simulink model "simulink10_3"  (R2025b)
settings: Solver=ode45  StartTime=0.0  StopTime=150.0  MaxStep=0.05  RelTol=1e-3
values from neighbouring files (symbols this model uses):
  C = Rs*Ps^-1    [lab10.m]
undefined symbols (not defined in the file or in its folder): A, B, D
settings Model: Creator=mizula  LastModifiedBy=mizula

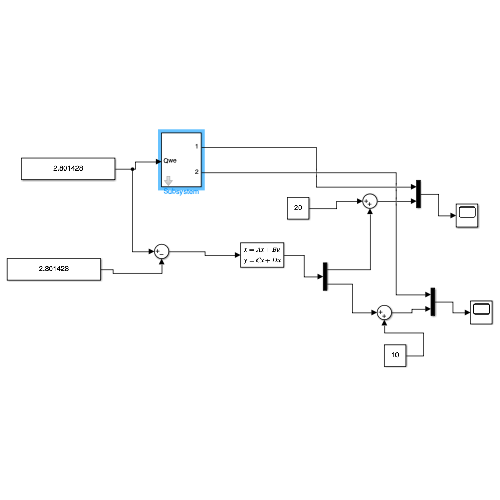
[thumbnail: Simulink's stored preview of the top-level diagram]
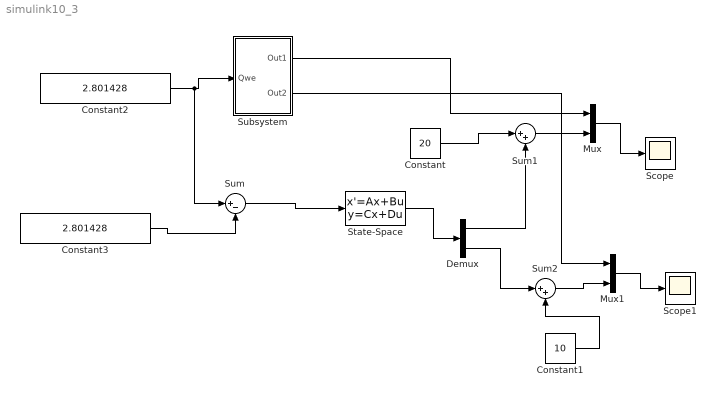
== system simulink10_3 ==
  Constant : Constant  Value=20
  Constant1 : Constant  Value=10
  Constant2 : Constant  Value=2.801428
  Constant3 : Constant  Value=2.801428
  Demux : Demux  Outputs=2
  Mux : Mux  Inputs=2
  Mux1 : Mux  Inputs=2
  Scope : Scope
      settings: ActiveDisplayYMinimum=-2.4999999999999996  ActiveDisplayYMaximum=22.5
  Scope1 : Scope
      settings: ActiveDisplayYMinimum=-1  ActiveDisplayYMaximum=1
  State-Space : StateSpace  A=A  B=B  C=C  D=D  InitialCondition=[0;0]
  Subsystem : Subsystem  mask{S1=1, S2=2, Swy1=0.2, Swy2=0.2, fi1=1, fi2=1, g=9.81, h1=20, h2=10}
  Sum : Sum  Inputs=|+-
  Sum1 : Sum  Inputs=|++
  Sum2 : Sum  Inputs=|++
  wires:
  Sum/1 -> State-Space/1
  Constant/1 -> Sum1/1
  Demux/1 -> Sum1/2
  State-Space/1 -> Demux/1
  Demux/2 -> Sum2/1
  Constant1/1 -> Sum2/2
  Sum1/1 -> Mux/2
  Subsystem/1(Out1) -> Mux/1
  Mux/1 -> Scope/1
  Sum2/1 -> Mux1/2
  Subsystem/2(Out2) -> Mux1/1
  Mux1/1 -> Scope1/1
  Constant2/1 -> Sum/1, Subsystem/1(Qwe)
  Constant3/1 -> Sum/2

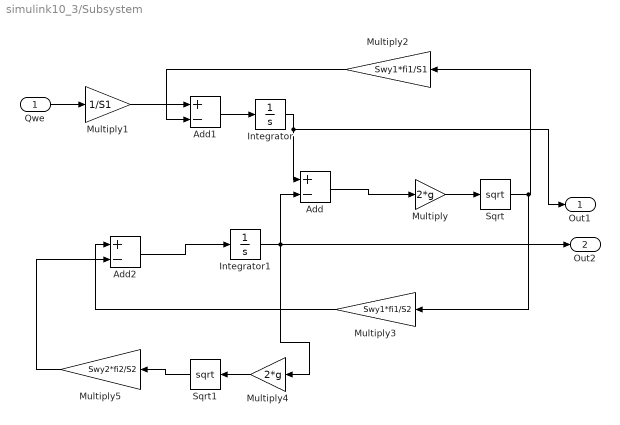
== system simulink10_3/Subsystem ==
  Qwe : Inport
  Add : Sum  Inputs=+-
  Add1 : Sum  Inputs=+-
  Add2 : Sum  Inputs=+-
  Integrator : Integrator  InitialCondition=h1
  Integrator1 : Integrator  InitialCondition=h2
  Multiply : Gain  Gain=2*g
  Multiply1 : Gain  Gain=1/S1
  Multiply2 : Gain  Gain=Swy1*fi1/S1
  Multiply3 : Gain  Gain=Swy1*fi1/S2
  Multiply4 : Gain  Gain=2*g
  Multiply5 : Gain  Gain=Swy2*fi2/S2
  Sqrt : Sqrt
  Sqrt1 : Sqrt
  Out1 : Outport
  Out2 : Outport  Port=2
  wires:
  Integrator1/1 -> Add/2, Multiply4/1, Out2/1
  Add/1 -> Multiply/1
  Integrator/1 -> Add/1, Out1/1
  Qwe/1 -> Multiply1/1
  Multiply4/1 -> Sqrt1/1
  Multiply5/1 -> Add2/2
  Multiply/1 -> Sqrt/1
  Sqrt/1 -> Multiply2/1, Multiply3/1
  Multiply1/1 -> Add1/1
  Add1/1 -> Integrator/1
  Sqrt1/1 -> Multiply5/1
  Add2/1 -> Integrator1/1
  Multiply2/1 -> Add1/2
  Multiply3/1 -> Add2/1
